simulink library "component_lib"  (R2023a)
settings: Solver=VariableStepAuto  StartTime=0.0  StopTime=10.0  RelTol=1e-3
undefined symbols (not defined in the file or in its folder): ECCV_r, par, R1234yf_ph, V_nom
libraries: base_lib x258, $bdroot x212, simulink x2, slpidlib x1
(part 3 of 7)

== system component_lib/Thermal Systems ==
  note: TitanX Radiator blockset
  RF0003_compressor : Subsystem  mask{V_disp=0.00017, N_ref=2000, t_c=1, W0=25e-3}
      mask prompts: V_disp "Displacement Volume [m3]:"; N_ref "Refrence Speed [rpm]:"; t_c "Compressor time constant [s]:"; W0 "Initial flow [kg/s]:"
      mask init:
      | % fluid properties
      | 
      | par = struct;
      | par.V_disp = V_disp;
      | par.N_ref  = N_ref;
      | 
      | setRefrigerantProperties;
  RF0004_smoothTube : Subsystem  mask{D=8e-3, L=1}
      mask prompts: D "Tube diameter [m]:"; L "Tube length [m]:"
      mask init:
      | % fluid properties
      | 
      | par = struct;
      | par.D = D;
      | par.L = L;
      | 
      | setRefrigerantProperties;
  RF0005_expansionValve : Subsystem  mask{D=1.8e-3, p_min=150e3}
      mask prompts: D "Orifice diameter [m]:"; p_min "Minimum Downstream Pressure [Pa]:"
      mask init:
      | % fluid properties
      | 
      | setRefrigerantProperties;
      | 
      | par.D = D;
  RF0007_PHEX : Subsystem  mask{N_ch=10, L=180e-3, B=65e-3, H=2e-3, t=0.3e-3, D_h=2.61e-3, N_nod=10, coolant_type=1}
      mask prompts: N_ch "Plates [-]:"; L "Length [m]:"; B "Width [m]:"; H "Height [m]:"; t "Plate thickness [m]"; D_h "Hydraulic Diameter [m]:"; N_nod "Nodes [even integer]"; coolant_type "Coolant type [-]:"
      mask init:
      | % fluid properties
      | 
      | setRefrigerantProperties;
      | 
      | par.type = coolant_type;
      | 
      | % Linearly spaced nodes
      | dx = L ./ N_nod;
      | 
      | % flow cross section area
      | A_c = H .* B;
      | 
      | % Volume per node
      | V = B .* H .* dx;
      | 
      | % aluminium properties
      | cp_w     = 0.9e3; % [J/kg K] specific heat
      | k_w      = 237;   % [W / mK] thermal conductivity
      | rho_w    = 2710;
      | A_w      = t .* B;
      | V_w      = t .* B .* dx;
      | d_w      = dx;
      | 
      | % hydraulic diameter
      | par.D_h = D_h;
      | 
      | % heat transfer area for each node
      | A =  B .* dx;
  RF0008_receiver_old : Subsystem  mask{V=1e-3, h0=280e3, p0=1e6, p_gain=1e3}
      mask prompts: V "Volume [m3]:"; h0 "Enthalpy [J/kg]:"; p0 "Pressure [Pa]:"; p_gain "Pressure gain:"
      mask init:
      | % fluid properties
      | par = struct;
      | setRefrigerantProperties;
      mask DialogControl Container4 Prompt: Parameters:
      mask DialogControl Container3 Prompt: Initial conditions:
      mask DialogControl Container5 Prompt: Relaxation Parameters:
  RF0010_calculateSuperHeat : Subsystem
      mask init:
      | % fluid properties
      | par = struct;
      | setRefrigerantProperties;
      mask DialogControl Container4 Prompt: Parameters:
  RF0011_calculateSubCool : Subsystem
      mask init:
      | % fluid properties
      | par = struct;
      | setRefrigerantProperties;
      mask DialogControl Container4 Prompt: Parameters:
  RF0012_louverFinHEX : Subsystem  mask{h00=400e3, N_tub=30, T_L=0.3, T_p=10.15e-3, T_d=16e-3, N_ch=18, a=1.3e-3, b=0.58e-3, L_a=23, F_p=1.4e-3, L_p=1.7e-3, L_l=6.4e-3, H=8.15e-3, d_f=16e-3, F_d=16e-3, N_nod=10}
      mask prompts: h00 "Enthalpy [J/kg]:"; N_tub "Nr. of Tubes [-]"; T_L "Tube length [m]:"; T_p "Tube pitch [m]:"; T_d "Tube depth [m]:"; N_ch "Minichannels per tube [-]"; a "Minichannel height [m]"; b "Minichannel width [m]"; L_a "Louver angle [deg]:"; F_p "Fin Pitch [m]:"; L_p "Louver Pitch [m]:"; L_l "Louver length [m]:"; H "Fin height [m]:"; d_f "Fin thickness [m]:"; F_d "Flow depth [m]:"; N_nod "Nodes [even integer]"
      mask init:
      | % fluid properties
      | 
      | setRefrigerantProperties;
      | setCoolantProperties;
      | setAirProperties;
      | 
      | % channel parameters
      | par.a = a;
      | par.b = b;
      | 
      | % Louver fin parameters
      | par.L_a  = L_a;  % Louver angle [deg]
      | par.F_p  = F_p;  % Fin pitch [m]
      | par.L_p  = L_p;  % Louver pitch [m]
      | par.L_l  = L_l;  % Louver length [m]
      | par.H    = H;    % Fin height [m]
      | par.T_p  = T_p;  % Tube pitch [m]
      | par.T_d  = T_d;  % Tube depth [m]
      | par.d_f  = d_f;  % Fin thickness [m]
      | par.F_d  = F_d;  % Flow depth [m]
      | 
      | % Aluminium properties
      | cp_w  = 0.9e3; % [J/kg K] specific heat
      | k_w   = 237;   % [W / mK] thermal conductivity
      | rho_w = 2710;
      | 
      | par.cp_w = cp_w;
      | par.k_w = k_w;
      | par.rho_w = rho_w;
      | 
      | 
      | % uniformly spaced nodes
      | dx = T_L ./ N_nod;
      | 
      | % Inner channel surface
      | A_wr = 2.*(a+b) .* dx .*  N_ch;
      | 
      | % Hydraulic diameter
      | D_h =  2 .* a .* b /(a + b);
      | par.D_h = D_h;
      | 
      | % Channel volume per node
      | V = N_ch .* a .* b .* dx;
      | 
      | % approximate number of fins between two tubes
      | n_fin = T_L./F_p;
      | 
      | % Fin surface area per node per tube
      | A_f =  L_l .* F_d .* n_fin ./ N_nod;
      | par.A_f = A_f;
      | 
      | % Tube surfae area per node
      | A_tub = 2 .* dx .* T_d;
      | 
      | % Total surface area per node
      | A_o = A_f + A_tub;
      | par.A_o = A_o;
      | 
      | % free flow cross section area per tube
      | A_fr = T_p .*  T_L;
      | 
      | % minimum cross section area per tube
      | A_min = H .* T_L  - atan( L_a * pi / 180 ) * L_p .* L_l;
      | 
      | % contraction ratio
      | par.sigma = A_fr ./ A_min;
      | 
      | % metal volume per node
      | V_w = (T_d .* (T_p - H)  - a.*b*N_ch ) * dx + A_f .* d_f; 
      | 
      | % node distance
      | d_w = dx;
      | A_w = (T_d .* (T_p - H)  - a.*b*N_ch );
      | 
      | % air volume per node
      | V_air = A_min .* F_d ./ N_nod;
      mask DialogControl Container6 Prompt: Initial Conditions
      mask DialogControl Container5 Prompt: Tube Geometry
      mask DialogControl Container4 Prompt: Fin Geometry
      mask DialogControl ParameterGroupVar Prompt: DIscretization:
  RF0013_calculateHeatflow : Subsystem
      mask init:
      | % fluid properties
      | par = struct;
      | setRefrigerantProperties;
      | setCoolantProperties;
      mask DialogControl Container4 Prompt: Parameters:
  RF0014_calculateVaporFraction : Subsystem
      mask init:
      | % fluid properties
      | par = struct;
      | setRefrigerantProperties;
      mask DialogControl Container4 Prompt: Parameters:
  RF0015_singlePhaseControlVolume : Subsystem  mask{V=1e-3, p0=200e3, h0=420e3}
      mask prompts: V "Volume [m3]"; p0 "Pressure [Pa]:"; h0 "Enthalpy [J/kg]:"
      mask init:
      | % fluid properties
      | par = struct;
      | setRefrigerantProperties;
      mask DialogControl Container4 Prompt: Parameters:
      mask DialogControl Container3 Prompt: Initial Conditions:
  RF0016_split : Subsystem
      mask init:
      | % fluid properties
      | 
      | 
      | setRefrigerantProperties;
  RF0017_merge : Subsystem  mask{V=1e-3}
      mask prompts: V "Volume [m3]:"
      mask init:
      | % fluid properties
      | 
      | 
      | setRefrigerantProperties;
  RF0018_calculateTemperature : Subsystem
      mask init:
      | % fluid properties
      | par = struct;
      | setRefrigerantProperties;
      mask DialogControl Container4 Prompt: Parameters:
  RF0019_receiver : Subsystem  mask{V=1e-3, h0=280e3, p0=1.6e6, p_gain=1e-3}
      mask prompts: V "Volume [m3]:"; h0 "Enthalpy [J/kg]:"; p0 "Pressure [Pa]:"; p_gain "Pressure gain:"
      mask init:
      | % fluid properties
      | par = struct;
      | setRefrigerantProperties;
      mask DialogControl Container4 Prompt: Parameters:
      mask DialogControl Container3 Prompt: Initial conditions:
      mask DialogControl Container5 Prompt: Relaxation Parameters:
  RF0020_simpleLouverFinHEX : Subsystem  mask{N_tub=30, T_L=0.3, T_p=10.15e-3, T_d=16e-3, N_ch=18, a=1.3e-3, b=0.58e-3, L_a=23, F_p=1.4e-3, L_p=1.7e-3, L_l=6.4e-3, H=8.15e-3, d_f=16e-3, F_d=16e-3}
      mask prompts: N_tub "Nr. of Tubes [-]"; T_L "Tube length [m]:"; T_p "Tube pitch [m]:"; T_d "Tube depth [m]:"; N_ch "Minichannels per tube [-]"; a "Minichannel height [m]"; b "Minichannel width [m]"; L_a "Louver angle [deg]:"; F_p "Fin Pitch [m]:"; L_p "Louver Pitch [m]:"; L_l "Louver length [m]:"; H "Fin height [m]:"; d_f "Fin thickness [m]:"; F_d "Flow depth [m]:"
      mask init:
      | % fluid properties
      | 
      | setRefrigerantProperties;
      | setCoolantProperties;
      | setAirProperties;
      | 
      | % channel parameters
      | par.a = a;
      | par.b = b;
      | 
      | % Louver fin parameters
      | par.L_a  = L_a;  % Louver angle [deg]
      | par.F_p  = F_p;  % Fin pitch [m]
      | par.L_p  = L_p;  % Louver pitch [m]
      | par.L_l  = L_l;  % Louver length [m]
      | par.H    = H;    % Fin height [m]
      | par.T_p  = T_p;  % Tube pitch [m]
      | par.T_d  = T_d;  % Tube depth [m]
      | par.d_f  = d_f;  % Fin thickness [m]
      | par.F_d  = F_d;  % Flow depth [m]
      | 
      | % Aluminium properties
      | cp_w  = 0.9e3; % [J/kg K] specific heat
      | k_w   = 237;   % [W / mK] thermal conductivity
      | rho_w = 2710;
      | 
      | par.cp_w = cp_w;
      | par.k_w = k_w;
      | par.rho_w = rho_w;
      | 
      | 
      | % Inner channel surface
      | A_wr = 2.*(a+b) .* T_L .*  N_ch;
      | 
      | % Hydraulic diameter
      | D_h =  2 .* a .* b /(a + b);
      | par.D_h = D_h;
      | 
      | % Channel volume
      | V = N_ch .* a .* b .* T_L;
      | 
      | % approximate number of fins between two tubes
      | n_fin = T_L./F_p;
      | 
      | % Fin surface area per tube
      | A_f =  L_l .* F_d .* n_fin;
      | par.A_f = A_f;
      | 
      | % Tube surfae area
      | A_tub = 2 .* T_L .* T_d;
      | 
      | % Total surface area per node
      | A_o = A_f + A_tub;
      | par.A_o = A_o;
      | 
      | % free flow cross section area per tube
      | A_fr = T_p .*  T_L;
      | 
      | % minimum cross section area per tube
      | A_min = H .* T_L  - atan( L_a * pi / 180 ) * L_p .* L_l;
      | 
      | % contraction ratio
      | par.sigma = A_fr ./ A_min;
      mask DialogControl Container5 Prompt: Tube Geometry
      mask DialogControl Container4 Prompt: Fin Geometry
  RF0021_simplePHEX : Subsystem  mask{N_ch=10, L=180e-3, B=65e-3, H=2e-3, t=0.3e-3, D_h=2.61e-3, coolant_type=1}
      mask prompts: N_ch "Plates [-]:"; L "Length [m]:"; B "Width [m]:"; H "Height [m]:"; t "Plate thickness [m]"; D_h "Hydraulic Diameter [m]:"; coolant_type "Coolant type [-]:"
      mask init:
      | % fluid properties
      | 
      | setRefrigerantProperties;
      | par.type = coolant_type;
      | 
      | 
      | % flow cross section area
      | A_c = H .* B;
      | 
      | % Volume
      | V = B .* H .* L;
      | 
      | % hydraulic diameter
      | par.D_h = D_h;
      | 
      | % heat transfer area
      | A =  B .* L; 
      | 
      | % aluminium properties
      | cp_w     = 0.9e3; % [J/kg K] specific heat
      | k_w      = 237;   % [W / mK] thermal conductivity
      | rho_w    = 2710;
      | A_w      = t .* B;
      | V_w      = t .* B .* L;
  RF0022_simpleExpansionValve : Subsystem  mask{D=1.8e-3, p_min=150e3, C=0.3}
      mask prompts: D "Orifice diameter [m]:"; p_min "Minimum Downstream Pressure [Pa]:"; C "Discharge coefficient [-]:"
      mask init:
      | % fluid properties
      | 
      | setRefrigerantProperties;
      | 
      | par.D = D;
      | par.C = C;
  RF0022_valve : Subsystem  mask{d=10e-2, dr=5e-2, C_d=0.9}
      mask prompts: d "Inlet port diameter [m]:"; dr "Restriction diameter [m]:"; C_d "Discharge coefficient [-]:"
      mask init:
      | % parameter struct
      | par = struct;
      | 
      | 
      | 
      | % get parameters
      | % par.d    = eval(get_param(gcb, 'd'));
      | % par.dr   = eval(get_param(gcb, 'dr'));
      | % par.C_d  = eval(get_param(gcb, 'C_d'));
      | 
      | par.d    = d;
      | par.dr   = dr;
      | par.C_d  = C_d;
      | 
      | 
      | % fluid properties
      | setRefrigerantProperties;
  TH0002_radiatorCore : Subsystem  mask{HtH=1.1, StS=0.95, radmodel=52 mm, coolant_type=1}
      mask prompts: HtH "Effective header to header [m]:"; StS "Effective sideplate to sideplate [m]:"; radmodel "Core depth [m]:"; coolant_type "Coolant type [-]:"
      mask init:
      | % parameter struct
      | par = struct;
      | 
      | % % get parameters
      | % par.HtH = eval(get_param(gcb, 'HtH'));
      | % par.StS = eval(get_param(gcb, 'StS'));
      | 
      | par.HtH = HtH;
      | par.StS = StS;
      | 
      | % Geometry
      | par.A_face = HtH * StS;
      | 
      | % Total heat transfer coefficient model:
      | par.cUexp = [0.7; 0.8];
      | 
      | switch radmodel
      |     
      |         case '19 mm'
      |         % Core depth
      |         par.CdT = 24e-3;
      |         
      |         % Heat trf. coefficient coefficients
      |         par.cU = [1.118075425066717e-04;
      |                   5.580064095289469e-04;
      |                   2.895685646303412e-05];
      |         
      |         % pressure drop coefficients
      |         par.c_dp_air = [37.253944105671480;
      |                          2.916659649936296e+02];         
      |         par.c_dp_clt = [19.727883408911566;
      |                          5.313528394369467];
      |         
      |         % relative area factors:
      |         rel_air = 0.752767994911226;
      |         rel_clt = 0.127946647958308;
      |     
      |     
      |         case '24 mm'
      |         % Core depth
      |         par.CdT = 24e-3;
      |         
      |         % Heat trf. coefficient coefficients
      |         par.cU = [9.815616404383520e-05;
      |                   4.676700861536502e-04;
      |                   2.415838699598361e-05];
      |         
      |         % pressure drop coefficients
      |         par.c_dp_air = [45.764851256613420;
      |                          2.404056250729179e+02];         
      |         par.c_dp_clt = [18.543378283094310;
      |                          5.151503273505832];
      |         
      |         % relative area factors:
      |         rel_air = 0.733387923444172;
      |         rel_clt = 0.132407142901122;
      |     
      |     
      |     
      |     case '42 mm'
      |         % Core depth
      |         par.CdT = 42e-3;
      |         
      |         % Heat trf. coefficient coefficients
      |         par.cU = [5.544027785616380e-05; 
      |                   2.449228920498670e-04; 
      |                   1.520415888705416e-05];
      |         
      |         % pressure drop coefficients
      |         par.c_dp_air = [36.973761781463810;
      |                          2.758340137219987e+02];
      |         par.c_dp_clt = [19.845956523612838;
      |                          5.112131585795914];
      |         
      |         % relative area factors:
      |         rel_air = 0.752767994911226;
      |         rel_clt = 0.115761252914660;
      |         
      |     case '52 mm'
      |         % Core depth
      |         par.CdT = 52e-3;
      |         
      |         % Heat trf. coefficient coefficients
      |         par.cU = [5.19516413772077e-05;
      |                   0.000198353781023090;
      |                   1.28249375163373e-05];
      |         
      |         % pressure drop coefficients
      |         par.c_dp_air = [46.462548129557995;
      |                          2.255631867184913e+02];
      |         par.c_dp_clt = [18.741626674634468;
      |                          4.871890188700768];
      |         
      |         % relative area factors:
      |         rel_air = 0.7334;
      |         rel_clt = 0.1222;
      | end
      | 
      | 
      | % Flow areas:
      | par.A_air  = rel_air * par.A_face; % Characteristic flow area
      | par.A_clt  = rel_clt * par.CdT * StS;  % Characteristic flow area
      | 
      | % fluid properties
      | % setCoolantProperties;
      | setAirProperties;
      | 
      | % coolant type
      | par.type = coolant_type;
      mask TypeOptions radmodel: 19 mm | 24 mm | 42 mm | 52 mm
  TH0003_coolantTank : Subsystem  mask{StS=0.95, D_con=0.055, T_0=273 + 25, radmodel=52 mm, coolant_type=1}
      mask prompts: StS "Sideplate to sideplate [m]"; D_con "Connector internal diameter [m]:"; T_0 "Temperature initial condition [K]:"; radmodel "Core depth [mm]:"; coolant_type "Coolant type [-]"
      mask init:
      | par = struct;
      | 
      | % fluid properties
      | % setCoolantProperties;
      | setAirProperties;
      | 
      | par.type = coolant_type;
      | 
      | 
      | % pressure drop coeffcient
      | par.zeta = 3;
      | 
      | % set core depth
      | switch radmodel
      |     
      |     case '19 mm'
      |         % Core depth
      |         par.CdT = 19e-3;
      |         
      |     case '24 mm'
      |         % Core depth
      |         par.CdT = 24e-3;
      |     
      |     case '42 mm'
      |         % Core depth
      |         par.CdT = 42e-3;
      |         
      |     case '52 mm'
      |         % Core depth
      |         par.CdT = 52e-3;
      | end
      | 
      | % Geometry
      | % tank volume
      | par.V = par.CdT.^2 * StS;
      | 
      | % inlet area
      | par.A_con = D_con.^2 .* pi/4;
      mask TypeOptions radmodel: 19 mm | 24 mm | 42 mm | 52 mm
  TH0004_radiatorPlugFlow : Subsystem  mask{HtH=1.1, StS=0.95, T_0=286, radmodel=52 mm, coolant_type=1}
      mask prompts: HtH "Header to header [m]:"; StS "Sideplate to sideplate [m]:"; T_0 "Temperature initial condition [K]:"; radmodel "Core depth [mm]:"; coolant_type "Coolant type [-]:"
      mask init:
      | par = struct;
      | 
      | % get parameters
      | % par.HtH = eval(get_param(gcb, 'HtH'));
      | % par.StS = eval(get_param(gcb, 'StS'));
      | 
      | par.HtH = HtH;
      | par.StS = StS;
      | 
      | % fluid properties
      | % setCoolantProperties;
      | setAirProperties;
      | 
      | par.type = coolant_type;
      | 
      | % set core depth
      | switch radmodel
      |     case '42 mm'
      |         % Core depth
      |         par.CdT = 42e-3;
      |         
      |     case '52 mm'
      |         % Core depth
      |         par.CdT = 52e-3;
      | end
      mask TypeOptions radmodel: 19 mm | 24 mm | 42 mm | 52 mm
  TH0005_flowSplit : Subsystem
      mask init:
      | % fluid properties
      | setCoolantProperties;
      | setAirProperties;
  TH0006_flowConfluence : Subsystem  mask{gain=0.01}
      mask prompts: gain "Flow balance gain [-]:"
      mask init:
      | % fluid properties
      | % setCoolantProperties;
      | setAirProperties;
  TH0007_airRestriction : Subsystem  mask{A=0.8, zeta=0.3}
      mask prompts: A "Area [m2]:"; zeta "Pressure drop coefficient [-]:"
      mask init:
      | % get parameters
      | % par.A    = eval(get_param(gcb, 'A'));
      | % par.zeta = eval(get_param(gcb, 'zeta'));
      | 
      | par.A    = A;
      | par.zeta = zeta;
      | 
      | % fluid properties
      | setAirProperties;
  TH0008_condenser : Subsystem  mask{HtH=0.85, StS=0.35, cdsmodel=16 mm}
      mask prompts: HtH "Header to header [m]:"; StS "Sideplate to sideplate [m]:"; cdsmodel "Core depth [m]:"
      mask init:
      | % parameter struct
      | par = struct;
      | 
      | % get parameters
      | % par.HtH = eval(get_param(gcb, 'HtH'));
      | % par.StS = eval(get_param(gcb, 'StS'));
      | 
      | par.HtH = HtH;
      | par.StS = StS;
      | 
      | 
      | switch cdsmodel
      |     case '16 mm'
      |         % Core depth
      |         par.CdT = 16-3;
      |         
      |         % pressure drop coefficients
      |         par.c_dp = [2.5; 6];
      |         
      |         
      |     case '18.8 mm'
      |         % Core depth
      |         par.CdT = 18.8e-3;
      |         
      |         % pressure drop coefficients
      |         par.c_dp = [2.7; 11];
      | end
      | 
      | % fluid properties
      | setAirProperties;
      mask TypeOptions cdsmodel: 16 mm | 18.8 mm
  TH0009_intake : Subsystem  mask{zeta=0.9}
      mask prompts: zeta "Pressure increase coefficient [-]:"
      mask init:
      | % get parameters
      | % par.zeta = eval(get_param(gcb, 'zeta'));
      | par.zeta = zeta;
      | 
      | % fluid properties
      | setAirProperties;
  TH0010_fan : Subsystem  mask{n_fan=4}
      mask prompts: n_fan "Nr. of fans [-]:"
      mask init:
      | % parameter struct
      | par = struct;
      | 
      | % get parameters
      | % par.n_fan = eval(get_param(gcb, 'n_fan'));
      | par.n_fan = n_fan;
      | 
      | 
      | % fan parameters
      | par.dpr   = -200;
      | par.q0    = 4290/3600;
      | par.dp0   = 800;
      | par.P_nom = 832;
      | 
      | 
      | % fluid properties
      | setAirProperties;
  TH0011_coolingChannel : Subsystem  mask{d=2e-3, L=50e-2, n_ch=1, e=0.006e-3, coolant_type=1}
      mask prompts: d "Hydraulic diameter [m]:"; L "Length [m]:"; n_ch "Nr. of channels [-]:"; e "Roughness [-]:"; coolant_type "Coolant type [-]"
      mask init:
      | % parameter struct
      | par = struct;
      | par.d = d;
      | par.L = L;
      | par.e = e;
      | 
      | % fluid properties
      | setAirProperties;
      | 
      | par.type = coolant_type
  TH0011_outletFlowBalance : Subsystem  mask{gain=0.05}
      mask prompts: gain "Dyn. balancing factor [m]:"
      mask init:
      | % fluid properties
      | setAirProperties;
  TH0011_pipe : Subsystem  mask{d=5e-2, L=1, e=0.006e-3, T_0=273 + 20, coolant_type=1}
      mask prompts: d "Diameter [m]:"; L "Length [m]:"; e "Roughness [m]:"; T_0 "Initial temperature [K]:"; coolant_type "Coolant type [-]:"
      mask init:
      | % parameter struct
      | par = struct;
      | 
      | % get parameters
      | % par.d = eval(get_param(gcb, 'd'));
      | % par.L = eval(get_param(gcb, 'L'));
      | 
      | par.d = d;
      | par.L = L;
      | par.e = e;
      | 
      | % fluid properties
      | setAirProperties;
      | 
      | par.type = coolant_type;
  TH0011_thermalMass : Subsystem  mask{m=34, cp=691, T_0=273 + 20}
      mask prompts: m "Mass [kg]:"; cp "Heat capacity [J/kgK]:"; T_0 "Initial temperature [K]:"
      mask init:
      | % fluid properties
      | setAirProperties;
  TH0012_equalSplitMerge : Subsystem  mask{n=1}
      mask prompts: n "Split/merge flow [-]"
      mask init:
      | % fluid properties
      | setCoolantProperties;
      | setAirProperties;
  TH0014_valve : Subsystem  mask{d=10e-2, dr=5e-2, C_d=0.9, coolant_type=1}
      mask prompts: d "Inlet port diameter [m]:"; dr "Restriction diameter [m]:"; C_d "Discharge coefficient [-]:"; coolant_type "Coolant type [-]:"
      mask init:
      | % parameter struct
      | par = struct;
      | 
      | % get parameters
      | % par.d    = eval(get_param(gcb, 'd'));
      | % par.dr   = eval(get_param(gcb, 'dr'));
      | % par.C_d  = eval(get_param(gcb, 'C_d'));
      | 
      | par.d    = d;
      | par.dr   = dr;
      | par.C_d  = C_d;
      | 
      | 
      | % fluid properties
      | setAirProperties;
      | 
      | par.type = coolant_type;
  TH0015_totalHeatTransfer : Subsystem  mask{T_max=273+100, T_min=273, coolant_type=1}
      mask prompts: T_max "Max. Temperature [K]:"; T_min "Min.Temperature [K]"; coolant_type "Coolant type [-]:"
      mask init:
      | % parameter struct
      | par = struct;
      | 
      | % fluid properties
      | setAirProperties;
      | 
      | par.type = coolant_type;
  TH0016_calculateHeatflow : Subsystem  mask{coolant_type=1}
      mask prompts: coolant_type "Coolant type [-]:"
      mask init:
      | % fluid properties
      | par = struct;
      | 
      | par.type = coolant_type;
      mask DialogControl Container4 Prompt: Parameters:
  TH0017_calculateHeatflow : Subsystem
      mask init:
      | % fluid properties
      | par = struct;
      | setRefrigerantProperties;
      | setAirProperties;
      mask DialogControl Container4 Prompt: Parameters:
  TH0018_PHEX : Subsystem  mask{N_ch=10, L=180e-3, B=65e-3, H=2e-3, t=0.3e-3, D_h=2.61e-3, N_nod=10, coolant_type=1}
      mask prompts: N_ch "Plates [-]:"; L "Length [m]:"; B "Width [m]:"; H "Height [m]:"; t "Plate thickness [m]"; D_h "Hydraulic Diameter [m]:"; N_nod "Nodes [even integer]"; coolant_type "Coolant type [-]:"
      mask init:
      | % fluid properties
      | 
      | setRefrigerantProperties;
      | 
      | par.type = coolant_type;
      | 
      | % Linearly spaced nodes
      | dx = L ./ N_nod;
      | 
      | % flow cross section area
      | A_c = H .* B;
      | 
      | % Volume per node
      | V = B .* H .* dx;
      | 
      | % aluminium properties
      | cp_w     = 0.9e3; % [J/kg K] specific heat
      | k_w      = 237;   % [W / mK] thermal conductivity
      | rho_w    = 2710;
      | A_w      = t .* B;
      | V_w      = t .* B .* dx;
      | d_w      = dx;
      | 
      | % hydraulic diameter
      | par.D_h = D_h;
      | 
      | % heat transfer area for each node
      | A =  2 .* B .* dx;
  TH0019_airTotalHeatTransfer : Subsystem  mask{T_min=273-40, T_max=273+140}
      mask prompts: T_min "Min. Temp. [K]"; T_max "Max. Temp[K]"
      mask init:
      | % parameter struct
      | par = struct;
      | 
      | % fluid properties
      | setAirProperties;
  TH0020_cm100hp : Subsystem  mask{coolant_type=1}
      mask prompts: coolant_type "Coolant type [-]:"
      mask init:
      | % parameter struct
      | par   = struct;
      | 
      | % fluid properties
      | setAirProperties;
      | 
      | par.type = coolant_type;
  TH0020_staticPressureDrop : Subsystem  mask{dp=1e4}
      mask prompts: dp "Pressure drop [Pa]:"
      mask init:
      | % parameter struct
      | par = struct;
      | 
      | % fluid properties
      | setCoolantProperties;
      | setAirProperties;
  TH0021_tank : Subsystem  mask{T0=273.15 + 80}
      mask prompts: T0 "Temperature [K]:"
      mask init:
      | % fluid properties
      | setAirProperties;
      mask DialogControl Container3 Prompt: Initial conditions:
  TH0022_restriction : Subsystem  mask{d=3.5e-3, C=0.8}
      mask prompts: d "Diameter [m]:"; C "Discharge coef. [-]"
      mask init:
      | % parameter struct
      | par = struct;
      | 
      | % get parameters
      | % par.d = eval(get_param(gcb, 'd'));
      | % par.L = eval(get_param(gcb, 'L'));
      | 
      | par.d = d;
      | par.C = C;
      | 
      | % fluid properties
      | setAirProperties;
  TH0023_WP120 : Subsystem
      mask init:
      | % parameter struct
      | par   = struct;
      | 
      | % fluid properties
      | setAirProperties;
  TH0024_WP150 : Subsystem  mask{n=1}
      mask prompts: n "Parallel pumps [-]"
      mask init:
      | % parameter struct
      | par   = struct;
      | 
      | % fluid properties
      | setAirProperties;
      settings: LibrarySourceBlock=component_lib/Thermal Systems/TH0023_WP120
  TH0025_VA164A : Subsystem  mask{n=1}
      mask prompts: n "Nr. of fans [-]:"
      mask init:
      | % parameter struct
      | par   = struct;
      | 
      | % fluid properties
      | setAirProperties;
      settings: LibrarySourceBlock=component_lib/Thermal Systems/TH0023_WP120
  TH0026_airVolume : Subsystem  mask{V=3, T0=273.15 + 25}
      mask prompts: V "Volume [m3]:"; T0 "Initial temperature [K]:"
      mask init:
      | % get parameters
      | 
      | % fluid properties
      | setAirProperties;
  TH0027_hvacFlap : Subsystem  mask{A=0.8, zeta=0.3}
      mask prompts: A "Open area [m2]:"; zeta "Pressure drop coefficient [-]:"
      mask init:
      | % get parameters
      | % par.A    = eval(get_param(gcb, 'A'));
      | % par.zeta = eval(get_param(gcb, 'zeta'));
      | 
      | par.A    = A;
      | par.zeta = zeta;
      | 
      | % fluid properties
      | setAirProperties;
  TH0028_VA195 : Subsystem  mask{n=1}
      mask prompts: n "Nr. of fans [-]:"
      mask init:
      | % parameter struct
      | par   = struct;
      | 
      | % fluid properties
      | setAirProperties;
      settings: LibrarySourceBlock=component_lib/Thermal Systems/TH0023_WP120
  TH0029_cabinConvection : Subsystem  mask{A=10}
      mask prompts: A "Area [m2]:"
      mask init:
      | % get parameters
      | 
      | % fluid properties
      | setAirProperties;
  TH0030_batteryPackConvection : Subsystem  mask{A=2*10, h=1}
      mask prompts: A "Area [m2]:"; h "HTC [W/m2K]"
      mask init:
      | % get parameters
      | 
      | % fluid properties
      | setAirProperties;
  TH0031_simplePHEX : Subsystem  mask{N_ch=10, L=180e-3, B=65e-3, H=2e-3, t=0.3e-3, D_h=2.61e-3, coolant_type=1}
      mask prompts: N_ch "Plates [-]:"; L "Length [m]:"; B "Width [m]:"; H "Height [m]:"; t "Plate thickness [m]"; D_h "Hydraulic Diameter [m]:"; coolant_type "Coolant type [-]:"
      mask init:
      | % fluid properties
      | 
      | setRefrigerantProperties;
      | 
      | par.type = coolant_type;
      | 
      | % Linearly spaced nodes
      | dx = L;
      | 
      | % flow cross section area
      | A_c = H .* B;
      | 
      | % Volume per node
      | V = B .* H .* dx;
      | 
      | % aluminium properties
      | cp_w     = 0.9e3; % [J/kg K] specific heat
      | k_w      = 237;   % [W / mK] thermal conductivity
      | rho_w    = 2710;
      | A_w      = t .* B;
      | V_w      = t .* B .* dx;
      | d_w      = dx;
      | 
      | % hydraulic diameter
      | par.D_h = D_h;
      | 
      | % heat transfer area for each node
      | A =  B .* dx;
  TH0032_VA113 : Subsystem  mask{n=1}
      mask prompts: n "Nr. of fans [-]:"
      mask init:
      | % parameter struct
      | par   = struct;
      | 
      | % fluid properties
      | setAirProperties;
      settings: LibrarySourceBlock=component_lib/Thermal Systems/TH0023_WP120

== system component_lib/Anode Gas Exchange/Subsystem1 ==
  W_an : Inport
  W_an_reacted : Inport  Port=2
  Demux : Demux
  Demux1 : Demux
  Divide : Product  Inputs=*/
  Gain : Gain  Gain=-1
  SC0002_signalRead11 : $bdroot/Data & Control/SC0002_signalRead  SigName=anodeStoichiometry
  Saturation : Saturate  UpperLimit=10  LowerLimit=-10
  wires:
  Divide/1 -> Saturation/1
  W_an/1 -> Demux/1
  Demux/1 -> Divide/1
  W_an_reacted/1 -> Gain/1
  Gain/1 -> Demux1/1
  Demux1/1 -> Divide/2
  Saturation/1 -> SC0002_signalRead11/1

== system component_lib/Cathode Gas Exchange/Subsystem1 ==
  W_ca : Inport
  W_ca_reacted : Inport  Port=2
  Demux : Demux
  Demux1 : Demux
  Divide : Product  Inputs=*/
  Gain : Gain  Gain=-1
  SC0002_signalRead11 : $bdroot/Data & Control/SC0002_signalRead  SigName=cathodeStoichiometry
  Saturation : Saturate  UpperLimit=10  LowerLimit=0
  wires:
  Divide/1 -> Saturation/1
  W_ca/1 -> Demux/1
  W_ca_reacted/1 -> Gain/1
  Gain/1 -> Demux1/1
  Saturation/1 -> SC0002_signalRead11/1
  Demux/2 -> Divide/1
  Demux1/2 -> Divide/2

== system component_lib/Data & Control/DC0007_cathodeFlowControl ==
  note: Oxygen flow [kg/s]
  note: Reference oxygen flow [kg/s]
  I_fc [A] : Inport
  W_ca [kg/s] : Inport  Port=2
  Cells in FC stack : Constant  Value=n_cell
  F0003_reactionFlow.m : base_lib/F0003_pukrushpan2004/F0003_reactionFlow.m  SystemSampleTime=-1  VariantActivationTime=update diagram  Latency=0  AutoFrameSizeCalculation=off
  Gain : Gain  Gain=1e5
  Gain1 : Gain  Gain=-1
  Oxygen mass fraction in dry air : Constant  Value=0.23
  Oxygen stoichiometry reference : Constant  Value=lambda_O2_ref
  PID Controller : slpidlib/PID Controller  Controller=PID  Form=Parallel  TimeDomain=Continuous-time  UseExternalTs=off  SampleTime=-1  IntegratorMethod=Forward Euler  FilterMethod=Forward Euler  ControllerParametersSource=internal  P=1  I=1  UseKiTs=off  D=0  N=100  UseFilter=on  TunerSelectOption=Transfer Function Based (PID Tuner App)  InitialConditionSource=internal  InitialConditionForIntegrator=0  InitialConditionForFilter=0  DifferentiatorICPrevScaledInput=0  ExternalReset=none  TrackingMode=off  Kt=1  LimitOutput=on  SatLimitsSource=internal  UpperSaturationLimit=2e4  LowerSaturationLimit=3e3  LinearizeAsGain=on  AntiWindupMode=back-calculation  Kb=1e-1  LimitIntegrator=off  UpperIntegratorSaturationLimit=inf  LowerIntegratorSaturationLimit=-inf  POutMin=[]  POutMax=[]  IOutMin=[]  IOutMax=[]  DOutMin=[]  DOutMax=[]  NOutMin=[]  NOutMax=[]  SumOutMin=[]  SumOutMax=[]  SaturationOutMin=[]  SaturationOutMax=[]  PParamMin=[]  PParamMax=[]  IParamMin=[]  IParamMax=[]  DParamMin=[]  DParamMax=[]  NParamMin=[]  NParamMax=[]  KbParamMin=[]  KbParamMax=[]  KtParamMin=[]  KtParamMax=[]  KbOutMin=[]  KbOutMax=[]  KtOutMin=[]  KtOutMax=[]  IntegratorOutMin=[]  IntegratorOutMax=[]  FilterOutMin=[]  FilterOutMax=[]  SumI1OutMin=[]  SumI1OutMax=[]  SumI2OutMin=[]  SumI2OutMax=[]  SumI3OutMin=[]  SumI3OutMax=[]  SumI4OutMin=[]  SumI4OutMax=[]  SumDOutMin=[]  SumDOutMax=[]  DifferentiatorOutMin=[]  DifferentiatorOutMax=[]  FilterDiffOutCoefMin=[]  FilterDiffOutCoefMax=[]  ReciprocalOutMin=[]  ReciprocalOutMax=[]  SumDenOutMin=[]  SumDenOutMax=[]  SumNumOutMin=[]  SumNumOutMax=[]  DivideOutMin=[]  DivideOutMax=[]  UdiffTsProdOutMin=[]  UdiffTsProdOutMax=[]  NTsProdOutMin=[]  NTsProdOutMax=[]  UintegralTsProdOutMin=[]  UintegralTsProdOutMax=[]  UngainTsProdOutMin=[]  UngainTsProdOutMax=[]  ClampingZeroOutDataTypeStr=Inherit: Inherit via back propagation  ClampingZeroOutMin=[]  ClampingZeroOutMax=[]  FilterDenConstantOutDataTypeStr=Inherit: Inherit via back propagation  FilterDenConstantOutMin=[]  FilterDenConstantOutMax=[]  PCopyOutDataTypeStr=Inherit: Inherit via back propagation  PCopyOutMin=[]  PCopyOutMax=[]  NCopyOutDataTypeStr=Inherit: Inherit via back propagation  NCopyOutMin=[]  NCopyOutMax=[]  IntegratorContinuousStateAttributes=''  IntegratorStateMustResolveToSignalObject=off  IntegratorRTWStateStorageClass=Auto  FilterContinuousStateAttributes=''  FilterStateMustResolveToSignalObject=off  FilterRTWStateStorageClass=Auto  ParallelPVariant=InternalParameters  IdealPVariant=Disabled  IVariant=InternalParameters  DVariant=InternalParameters  IntegratorVariant=Continuous  SatVariant=Enabled  AWVariant=BackCalculation  PCopyVariant=Disabled  TRVariant=Disabled  FdbkBlocksVariant=Forward  IdealPFdbkVariant=Disabled  SatFdbkVariant=Disabled  DerivativeFilterVariant=ContFilter  NVariant=InternalParameters  NCopyVariant=Disabled  FilterICVariant=InternalICsFilter  IntegratorICVariant=InternalICs  ExternalResetVariant=Disabled  TRSumVariant=Passthrough  SumFdbkVariant=Disabled  SumVariant=Sum_PID  TsampFilterVariant=InternalTs  TsampNgainVariant=Passthrough  TsampIntegralVariant=Passthrough  ExternalSaturationOutDataTypeStr=Inherit: Same as second input
  Product : Product  Inputs=3
  Product1 : Product
  Selector : Selector  InputPortWidth=4  IndexOptions=Index vector (dialog)  Indices=2  OutputSizes=1
  Sum : Sum  Inputs=|+-
  Terminator : Terminator
  w_cmp [rad/s] : Outport
  wires:
  F0003_reactionFlow.m/2 -> Selector/1
  Oxygen stoichiometry reference/1 -> Product/1
  Selector/1 -> Gain1/1
  Oxygen mass fraction in dry air/1 -> Product1/2
  F0003_reactionFlow.m/1 -> Terminator/1
  Gain1/1 -> Product/3
  Cells in FC stack/1 -> Product/2
  Product/1 -> Sum/1
  Product1/1 -> Sum/2
  Sum/1 -> Gain/1
  PID Controller/1 -> w_cmp [rad/s]/1
  Gain/1 -> PID Controller/1
  I_fc [A]/1 -> F0003_reactionFlow.m/1
  W_ca [kg/s]/1 -> Product1/1

== system component_lib/Data & Control/DC0008_linearMPCSolver ==
  A [n x n] : Inport
  B [n x m] : Inport  Port=2
  Constant : Constant  Value=Q
  Constant1 : Constant  Value=R
  Constant2 : Constant  Value=N
  MPCtoQP : MATLAB Function  TreatAsAtomicUnit=on
  qpSWIFT : S-Function  FunctionName=qpSWIFT_sfunc_e  SFunctionDeploymentMode=off  EnableBusSupport=off
  u [ N x 1] : Outport
  exitFlag [-] : Outport  Port=2
  wires:
  A [n x n]/1 -> MPCtoQP/1(A)
  B [n x m]/1 -> MPCtoQP/2(B)
  Constant/1 -> MPCtoQP/3(Q)
  Constant1/1 -> MPCtoQP/4(R)
  Constant2/1 -> MPCtoQP/5(N)

== system component_lib/Data & Control/SC0002_signalRead ==
  SigIdentifier : Inport
  tag scope: SigIdentifier=global
  wires:
  SigIdentifier/1 -> [SigIdentifier]

== system component_lib/Data & Control/SC0003_signalWrite ==
  y : Outport
  wires:
  [SigIdentifier] -> y/1

== system component_lib/Electrochemistry/EL0001_panasonicNCR18650PF ==
  note: Kelvin -> degC
  I [A] : Inport
  T [K] : Inport  Port=2
  Abs : Abs  SaturateOnIntegerOverflow=off
  Constant : Constant  Value=273.15
  Constant5 : Constant  Value=3.6e3
  Divide1 : Product  Inputs=*//
  F0001_cellCapacity.m : base_lib/F0001_panasonicCell/F0001_cellCapacity.m  SystemSampleTime=-1  VariantActivationTime=update diagram  Latency=0  AutoFrameSizeCalculation=off
  F0001_dynamicVoltage.m : base_lib/F0001_panasonicCell/F0001_dynamicVoltage.m  SystemSampleTime=-1  VariantActivationTime=update diagram  Latency=0  AutoFrameSizeCalculation=off
  F0001_ocvSOC.m : base_lib/F0001_panasonicCell/F0001_ocvSOC.m  SystemSampleTime=-1  VariantActivationTime=update diagram  Latency=0  AutoFrameSizeCalculation=off
  Gain : Gain  Gain=-1
  Integrator Limited : Integrator  InitialCondition=par.init_SOC  LimitOutput=on  UpperSaturationLimit=1  LowerSaturationLimit=0
  Integrator1 : Integrator  InitialCondition=zeros(5,1)
  Product : Product
  Saturation : Saturate  UpperLimit=0.9  LowerLimit=0.1
  Sum : Sum  Inputs=|+-
  Sum2 : Sum  Inputs=|+-
  V [V] : Outport
  SOC [-] : Outport  Port=2
  Q_gen [J/s] : Outport  Port=3
  wires:
  F0001_dynamicVoltage.m/1 -> Integrator1/1
  Integrator1/1 -> F0001_dynamicVoltage.m/1
  T [K]/1 -> Sum2/1
  F0001_ocvSOC.m/1 -> Sum/1
  Integrator Limited/1 -> SOC [-]/1, Saturation/1
  Constant/1 -> Sum2/2
  Sum2/1 -> F0001_dynamicVoltage.m/2, F0001_cellCapacity.m/1
  Constant5/1 -> Divide1/2
  F0001_cellCapacity.m/1 -> Divide1/3
  Gain/1 -> Divide1/1
  Divide1/1 -> Integrator Limited/1
  Saturation/1 -> F0001_ocvSOC.m/1
  F0001_dynamicVoltage.m/2 -> Product/1, Sum/2
  Sum/1 -> V [V]/1
  Abs/1 -> Q_gen [J/s]/1
  Product/1 -> Abs/1
  I [A]/1 -> F0001_dynamicVoltage.m/3, Gain/1, Product/2

== system component_lib/Electrochemistry/EL0004_buckCCM ==
  V_in [V] : Inport
  I_out [A] : Inport  Port=2
  d [-] : Inport  Port=3
  Abs : Abs  SaturateOnIntegerOverflow=off
  Gain2 : Gain  Gain=1/C
  Gain4 : Gain  Gain=1/L
  Gain6 : Gain  Gain=R
  Integrator : Integrator
  Product{,1..3} (4 alike) : Product
  Saturation1 : Saturate  UpperLimit=1  LowerLimit=0
  Sum : Sum  Inputs=+|-
  Sum1 : Sum  Inputs=-+|
  Sum3 : Sum  Inputs=+-|
  Sum4 : Sum  Inputs=|++
  Transfer Fcn : TransferFcn  Denominator=[0.001 1]
  V_4 : Integrator  InitialCondition=V_init
  V_out [V] : Outport
  I_in [A] : Outport  Port=2
  Q_gen [J/s] : Outport  Port=3
  wires:
  Abs/1 -> Q_gen [J/s]/1
  Gain4/1 -> Integrator/1
  Gain6/1 -> Sum4/2
  Sum4/1 -> Sum1/1
  Sum1/1 -> Gain4/1
  Gain2/1 -> V_4/1
  Sum3/1 -> Gain2/1
  I_out [A]/1 -> [I_out], Sum3/2
  d [-]/1 -> Saturation1/1
  Integrator/1 -> Product/1, Gain6/1, Sum3/1
  Product1/1 -> Sum1/2
  Saturation1/1 -> Product1/2, Product/2
  Product/1 -> Transfer Fcn/1
  [I_out] -> Product2/2
  Sum/1 -> Abs/1
  V_in [V]/1 -> Product3/2, Product1/1
  Product3/1 -> Sum/2
  Product2/1 -> Sum/1
  V_4/1 -> Product2/1, V_out [V]/1, Sum4/1
  Transfer Fcn/1 -> Product3/1, I_in [A]/1

== system component_lib/Electrochemistry/EL0005_boostCCM ==
  note: Efficiency
  V_in [V] : Inport
  d [-] : Inport  Port=2
  I_out [A] : Inport  Port=3
  Abs : Abs  SaturateOnIntegerOverflow=off
  Add : Sum  Inputs=+-
  Add1 : Sum  Inputs=+-
  Add2 : Sum  Inputs=+--
  Capacitor voltage : Integrator  InitialCondition=V_init
  Constant : Constant
  Constant1 : Constant  Value=eta
  Divide1 : Product  Inputs=**
  Gain : Gain  Gain=1/L
  Gain1 : Gain  Gain=1/C
  Gain2 : Gain  Gain=-1
  Integrator : Integrator
  Power : Math  Operator=pow
  Product{,1..3} (4 alike) : Product
  Resistor to ground : Gain  Gain=1e-4
  Saturation : Saturate  UpperLimit=0.8  LowerLimit=0.2
  Sign : Signum
  Sum : Sum  Inputs=+|-
  Transfer Fcn : TransferFcn  Denominator=[0.001 1]
  V_out [V] : Outport
  I_in [A] : Outport  Port=2
  Q_gen [J/s] : Outport  Port=3
  wires:
  Divide1/1 -> I_in [A]/1, [I_in], Gain2/1
  Abs/1 -> Q_gen [J/s]/1
  Sum/1 -> Abs/1
  [V_out] -> Product2/1
  [V_in] -> Product3/1
  [I_out] -> Product2/2
  [I_in] -> Product3/2
  Product2/1 -> Sum/1
  Product3/1 -> Sum/2
  Power/1 -> Divide1/2
  Transfer Fcn/1 -> Sign/1
  Gain2/1 -> Transfer Fcn/1
  Sign/1 -> Power/2
  Constant1/1 -> Power/1
  Resistor to ground/1 -> Add2/3
  V_in [V]/1 -> Add1/1, [V_in]
  d [-]/1 -> Saturation/1
  I_out [A]/1 -> Add2/2, [I_out]
  Gain1/1 -> Capacitor voltage/1
  Add2/1 -> Gain1/1
  Product1/1 -> Add2/1
  Integrator/1 -> Product1/1, Divide1/1
  Add1/1 -> Gain/1
  Product/1 -> Add1/2
  Add/1 -> Product1/2, Product/1
  Gain/1 -> Integrator/1
  Capacitor voltage/1 -> V_out [V]/1, [V_out], Product/2, Resistor to ground/1
  Constant/1 -> Add/1
  Saturation/1 -> Add/2

== system component_lib/Electrochemistry/EL0006_busDC ==
  V_1 [V] : Inport
  I_load [A] : Inport  Port=2
  V_2 [V] : Inport  Port=3
  Gain : Gain  Gain=1/C
  Gain1 : Gain  Gain=1e-3
  Gain2 : Gain  Gain=1/L
  Gain3 : Gain  Gain=1/L
  Gain4 : Gain  Gain=R
  Gain6 : Gain  Gain=R
  Integrator : Integrator
  Integrator1 : Integrator
  Sum : Sum  Inputs=|+-
  Sum1 : Sum  Inputs=-+|
  Sum2 : Sum  Inputs=|+-
  Sum3 : Sum  Inputs=+-+
  Sum4 : Sum  Inputs=|++
  Sum5 : Sum  Inputs=++|
  V_4 : Integrator  InitialCondition=V_init
  I_1 [A] : Outport
  V_bus [V] : Outport  Port=2
  I_2 [A] : Outport  Port=3
  wires:
  Gain1/1 -> Sum/2
  Sum/1 -> Gain/1
  Sum3/1 -> Sum/1
  V_4/1 -> V_bus [V]/1, Sum5/2, Gain1/1, Sum4/1
  I_load [A]/1 -> Sum3/2
  Gain/1 -> V_4/1
  Integrator/1 -> I_1 [A]/1, Gain4/1, Sum3/1
  Integrator1/1 -> I_2 [A]/1, Gain6/1, Sum3/3
  Sum1/1 -> Gain2/1
  V_1 [V]/1 -> Sum1/2
  Sum2/1 -> Gain3/1
  V_2 [V]/1 -> Sum2/1
  Gain2/1 -> Integrator/1
  Gain3/1 -> Integrator1/1
  Gain4/1 -> Sum4/2
  Sum4/1 -> Sum1/1
  Gain6/1 -> Sum5/1
  Sum5/1 -> Sum2/2

== system component_lib/Electrochemistry/EL0007_pukrushpan2004 ==
  I [A] : Inport
  p_an [Pa x 4] : Inport  Port=2
  p_ca [Pa x 4] : Inport  Port=3
  T_an [K] : Inport  Port=4
  T_ca [K] : Inport  Port=5
  T_fc [K] : Inport  Port=6
  Demux : Demux
  Demux1 : Demux
  F0003_diffusiveFlow.m : base_lib/F0003_pukrushpan2004/F0003_diffusiveFlow.m  SystemSampleTime=-1  VariantActivationTime=update diagram  Latency=0  AutoFrameSizeCalculation=off
      settings: LibrarySourceBlock=|
      | simulink/User-Defined
      | Functions/MATLAB Function
  F0003_dragFlow.m : base_lib/F0003_pukrushpan2004/F0003_dragFlow.m  SystemSampleTime=-1  VariantActivationTime=update diagram  Latency=0  AutoFrameSizeCalculation=off
      settings: LibrarySourceBlock=|
      | simulink/User-Defined
      | Functions/MATLAB Function
  F0003_outputVoltage.m : base_lib/F0003_pukrushpan2004/F0003_outputVoltage.m  SystemSampleTime=-1  VariantActivationTime=update diagram  Latency=0  AutoFrameSizeCalculation=off
      settings: LibrarySourceBlock=|
      | simulink/User-Defined
      | Functions/MATLAB Function
  F0003_reactionFlow.m : base_lib/F0003_pukrushpan2004/F0003_reactionFlow.m  SystemSampleTime=-1  VariantActivationTime=update diagram  Latency=0  AutoFrameSizeCalculation=off
      settings: LibrarySourceBlock=|
      | simulink/User-Defined
      | Functions/MATLAB Function
  F0003_vaporActivity.m : base_lib/F0003_pukrushpan2004/F0003_vaporActivity.m  SystemSampleTime=-1  VariantActivationTime=update diagram  Latency=0  AutoFrameSizeCalculation=off
      settings: LibrarySourceBlock=|
      | simulink/User-Defined
      | Functions/MATLAB Function
  F0003_vaporActivity.m1 : base_lib/F0003_pukrushpan2004/F0003_vaporActivity.m  SystemSampleTime=-1  VariantActivationTime=update diagram  Latency=0  AutoFrameSizeCalculation=off
      settings: LibrarySourceBlock=|
      | simulink/User-Defined
      | Functions/MATLAB Function
  F0003_waterContent.m : base_lib/F0003_pukrushpan2004/F0003_waterContent.m  SystemSampleTime=-1  VariantActivationTime=update diagram  Latency=0  AutoFrameSizeCalculation=off
      settings: LibrarySourceBlock=|
      | simulink/User-Defined
      | Functions/MATLAB Function
  F0003_waterContent.m1 : base_lib/F0003_pukrushpan2004/F0003_waterContent.m  SystemSampleTime=-1  VariantActivationTime=update diagram  Latency=0  AutoFrameSizeCalculation=off
      settings: LibrarySourceBlock=|
      | simulink/User-Defined
      | Functions/MATLAB Function
  F0010_vaporSaturationPressure.m : base_lib/F0010_gasFlow/F0010_vaporSaturationPressure.m  SystemSampleTime=-1  VariantActivationTime=update diagram  Latency=0  AutoFrameSizeCalculation=off
      settings: LibrarySourceBlock=|
      | simulink/User-Defined
      | Functions/MATLAB Function
  F0010_vaporSaturationPressure.m1 : base_lib/F0010_gasFlow/F0010_vaporSaturationPressure.m  SystemSampleTime=-1  VariantActivationTime=update diagram  Latency=0  AutoFrameSizeCalculation=off
      settings: LibrarySourceBlock=|
      | simulink/User-Defined
      | Functions/MATLAB Function
  F0010_vaporSaturationPressure.m2 : base_lib/F0010_gasFlow/F0010_vaporSaturationPressure.m  SystemSampleTime=-1  VariantActivationTime=update diagram  Latency=0  AutoFrameSizeCalculation=off
      settings: LibrarySourceBlock=|
      | simulink/User-Defined
      | Functions/MATLAB Function
  Gain : Gain  Gain=1/2
  Mux : Mux
  Saturation : Saturate  UpperLimit=inf  LowerLimit=0.01
  Saturation1 : Saturate  UpperLimit=inf  LowerLimit=100
  Saturation2 : Saturate  UpperLimit=inf  LowerLimit=100
  Sum : Sum  Inputs=+|+
  Sum1 : Sum  Inputs=|+-
  Sum2 : Sum  Inputs=|++
  Sum4 : Sum  Inputs=|++
  V [V] : Outport
  W_an [kg/s] : Outport  Port=2
  W_ca [kg/s] : Outport  Port=3
  lam [-] : Outport  Port=4
  Q_gen [J/s] : Outport  Port=5
  wires:
  I [A]/1 -> [I], F0003_reactionFlow.m/1, F0003_outputVoltage.m/1
  F0003_outputVoltage.m/1 -> Saturation/1
  F0003_outputVoltage.m/2 -> Q_gen [J/s]/1
  T_fc [K]/1 -> F0003_diffusiveFlow.m/4, F0010_vaporSaturationPressure.m2/1, F0003_outputVoltage.m/6
  F0010_vaporSaturationPressure.m2/1 -> F0003_outputVoltage.m/4
  F0010_vaporSaturationPressure.m1/1 -> F0003_vaporActivity.m/2
  F0010_vaporSaturationPressure.m/1 -> F0003_vaporActivity.m1/2
  T_an [K]/1 -> F0010_vaporSaturationPressure.m1/1
  T_ca [K]/1 -> F0010_vaporSaturationPressure.m/1
  Demux/3 -> F0003_vaporActivity.m/1
  Demux1/3 -> F0003_vaporActivity.m1/1
  p_an [Pa x 4]/1 -> Demux/1, Saturation1/1
  p_ca [Pa x 4]/1 -> Demux1/1, Saturation2/1
  F0003_vaporActivity.m/1 -> F0003_waterContent.m/1
  F0003_vaporActivity.m1/1 -> F0003_waterContent.m1/1
  F0003_waterContent.m/1 -> Sum/1, F0003_diffusiveFlow.m/1
  F0003_waterContent.m1/1 -> F0003_diffusiveFlow.m/3, Sum/2
  F0003_reactionFlow.m/1 -> Sum1/1
  Sum1/1 -> W_an [kg/s]/1
  F0003_reactionFlow.m/2 -> Sum2/1
  Sum2/1 -> W_ca [kg/s]/1
  [I] -> F0003_dragFlow.m/1
  F0003_diffusiveFlow.m/1 -> Sum4/1
  F0003_dragFlow.m/1 -> Sum4/2
  Mux/1 -> Sum1/2, Sum2/2
  Sum/1 -> Gain/1
  Sum4/1 -> Mux/3
  Saturation/1 -> V [V]/1
  Saturation1/1 -> F0003_outputVoltage.m/2
  Saturation2/1 -> F0003_outputVoltage.m/3
  Gain/1 -> lam [-]/1, F0003_outputVoltage.m/5, F0003_dragFlow.m/2, F0003_diffusiveFlow.m/2

== system component_lib/Electrochemistry/EL0008_dcdcConverter ==
  I_in [A] : Inport
  V_in [V] : Inport  Port=2
  V_bus [V] : Inport  Port=3
  F0020_dcdcConverter.m : base_lib/F0020_dcdcConverter/F0020_dcdcConverter.m  SystemSampleTime=-1  VariantActivationTime=update diagram  Latency=0  AutoFrameSizeCalculation=off
      settings: LibrarySourceBlock=|
      | simulink/User-Defined
      | Functions/MATLAB Function
  Terminator : Terminator
  Terminator1 : Terminator
  I_bus [A] : Outport
  Q_gen [J/s] : Outport  Port=2
  wires:
  V_bus [V]/1 -> F0020_dcdcConverter.m/1
  V_in [V]/1 -> F0020_dcdcConverter.m/2
  I_in [A]/1 -> F0020_dcdcConverter.m/3
  F0020_dcdcConverter.m/2 -> I_bus [A]/1
  F0020_dcdcConverter.m/1 -> Terminator/1
  F0020_dcdcConverter.m/4 -> Q_gen [J/s]/1
  F0020_dcdcConverter.m/3 -> Terminator1/1

== system component_lib/Electrochemistry/EL0010_superCapacitor ==
  dI [A] : Inport
  Gain : Gain  Gain=1/C
  Integrator Limited : Integrator  InitialCondition=V_bus0  LimitOutput=on  LowerSaturationLimit=0
  V_bus [V] : Outport
  wires:
  Integrator Limited/1 -> V_bus [V]/1
  dI [A]/1 -> Gain/1
  Gain/1 -> Integrator Limited/1

== system component_lib/Electrochemistry/EL0011_ITPEMFC ==
  I [A] : Inport
  p_O2 [Pa] : Inport  Port=2
  T [K] : Inport  Port=3
  RH [-] : Inport  Port=4
  F0003_reactionFlow.m : base_lib/F0003_pukrushpan2004/F0003_reactionFlow.m  SystemSampleTime=-1  VariantActivationTime=update diagram  Latency=0  AutoFrameSizeCalculation=off
      settings: LibrarySourceBlock=|
      | simulink/User-Defined
      | Functions/MATLAB Function
  F0031_ITPEMFC.m : base_lib/F0031_ITPEMFC/F0031_ITPEMFC.m  SystemSampleTime=-1  VariantActivationTime=update diagram  Latency=0  AutoFrameSizeCalculation=off
      settings: LibrarySourceBlock=|
      | simulink/User-Defined
      | Functions/MATLAB Function
  Saturation : Saturate  UpperLimit=inf  LowerLimit=0.01
  V [V] : Outport
  W_an [kg/s] : Outport  Port=2
  W_ca [kg/s] : Outport  Port=3
  Q_gen [J/s] : Outport  Port=4
  wires:
  I [A]/1 -> F0003_reactionFlow.m/1, F0031_ITPEMFC.m/1
  F0031_ITPEMFC.m/1 -> Saturation/1
  F0031_ITPEMFC.m/2 -> Q_gen [J/s]/1
  F0003_reactionFlow.m/1 -> W_an [kg/s]/1
  F0003_reactionFlow.m/2 -> W_ca [kg/s]/1
  Saturation/1 -> V [V]/1
  p_O2 [Pa]/1 -> F0031_ITPEMFC.m/2
  T [K]/1 -> F0031_ITPEMFC.m/3
  RH [-]/1 -> F0031_ITPEMFC.m/4
